simulink model "P_2_1_i_Tempomat_modell"  (R2021b)
settings: Solver=VariableStepAuto  StartTime=0.0  StopTime=10  RelTol=1e-3
settings Model: Creator=davidpaksi  LastModifiedBy=davidpaksi

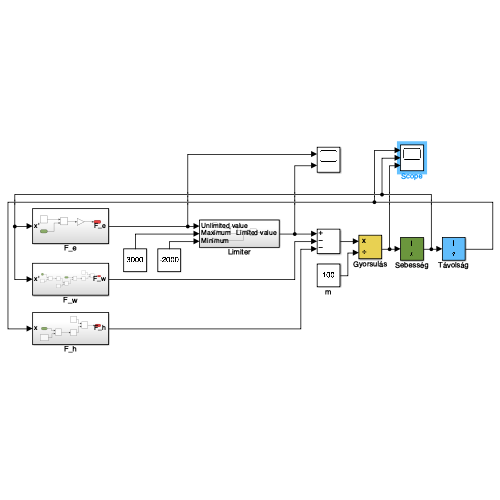
[thumbnail: Simulink's stored preview of the top-level diagram]
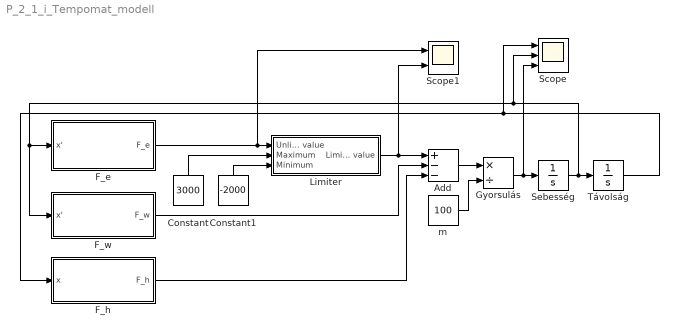
== system P_2_1_i_Tempomat_modell ==
  Add : Sum  Inputs=+--
  Constant : Constant  Value=3000
  Constant1 : Constant  Value=-2000
  F_e : Subsystem
  F_h : Subsystem
  F_w : Subsystem
  Gyorsulás : Product  Inputs=*/
  Limiter : Subsystem
  Scope : Scope  NumInputPorts=3
  Scope1 : Scope  NumInputPorts=2
  Sebesség : Integrator
  Távolság : Integrator
  m : Constant  Value=100
  wires:
  Sebesség/1 -> F_w/1(x'), F_e/1(x'), Scope/2, Távolság/1
  Gyorsulás/1 -> Scope/3, Sebesség/1
  m/1 -> Gyorsulás/2
  Add/1 -> Gyorsulás/1
  F_w/1(F_w) -> Add/2
  F_h/1(F_h) -> Add/3
  Távolság/1 -> Scope/1, F_h/1(x)
  F_e/1(F_e) -> Scope1/1, Limiter/1(Unlimited value)
  Limiter/1(Limited value) -> Scope1/2, Add/1
  Constant/1 -> Limiter/2(Maximum)
  Constant1/1 -> Limiter/3(Minimum)

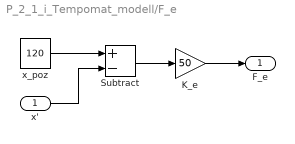
== system P_2_1_i_Tempomat_modell/F_e ==
  x' : Inport
  K_e : Gain  Gain=50
  Subtract : Sum  Inputs=+-
  x_poz : Constant  Value=120
  F_e : Outport
  wires:
  x'/1 -> Subtract/2
  x_poz/1 -> Subtract/1
  Subtract/1 -> K_e/1
  K_e/1 -> F_e/1

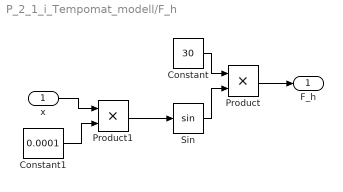
== system P_2_1_i_Tempomat_modell/F_h ==
  x : Inport
  " Sin " : Trigonometry
  Constant : Constant  Value=30
  Constant1 : Constant  Value=0.0001
  Product : Product
  Product1 : Product
  F_h : Outport
  wires:
  Product/1 -> F_h/1
  Constant/1 -> Product/1
  " Sin "/1 -> Product/2
  Product1/1 -> " Sin "/1
  Constant1/1 -> Product1/2
  x/1 -> Product1/1

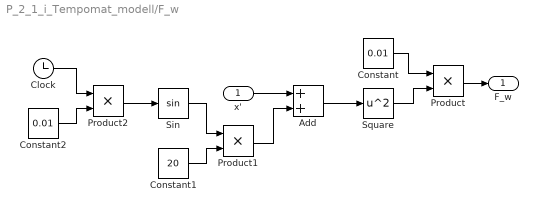
== system P_2_1_i_Tempomat_modell/F_w ==
  x' : Inport
  "  Clock " : Clock
  " Sin " : Trigonometry
  " Square " : Math  Operator=square  SaturateOnIntegerOverflow=on
  Add : Sum
  Constant : Constant  Value=0.01
  Constant1 : Constant  Value=20
  Constant2 : Constant  Value=0.01
  Product : Product
  Product1 : Product
  Product2 : Product
  F_w : Outport
  wires:
  Product/1 -> F_w/1
  Constant/1 -> Product/1
  " Square "/1 -> Product/2
  Add/1 -> " Square "/1
  x'/1 -> Add/1
  Product1/1 -> Add/2
  Constant1/1 -> Product1/2
  " Sin "/1 -> Product1/1
  Product2/1 -> " Sin "/1
  Constant2/1 -> Product2/2
  "  Clock "/1 -> Product2/1

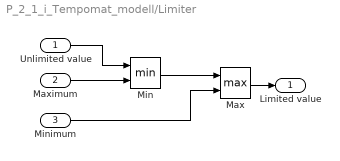
== system P_2_1_i_Tempomat_modell/Limiter ==
  Unlimited value : Inport
  Maximum : Inport  Port=2
  Minimum : Inport  Port=3
  Max : MinMax  Function=max  Inputs=2
  Min : MinMax  Inputs=2
  Limited value : Outport
  wires:
  Maximum/1 -> Min/2
  Unlimited value/1 -> Min/1
  Min/1 -> Max/1
  Minimum/1 -> Max/2
  Max/1 -> Limited value/1
